simulink model "Boat_sim_HeadingHold"  (Simulink 7.5)
settings: Solver=FixedStepDiscrete  StartTime=0.0  StopTime=1000  FixedStep=.01  RelTol=1e-3
InitFcn:
  | boat_constants
values from neighbouring files (symbols this model uses):
  C_d_sea_surge = 340    [boat_constants.m]
  d_prop = .4572    (= 0.4572)    [boat_constants.m]
  figure8_waypoints = int32([ ... (first row only)    [boat_constants.m]
  K_t = 0.5    [boat_constants.m]
  mass = 550    [boat_constants.m]
  OC2max = 49999    [boat_constants.m]    (also in simulation_constants.m)
  phi_0 = 0    [boat_constants.m]    (also in simulation_constants.m)
  rho_w = 1.03e3    (= 1030)    [boat_constants.m]
  sampling_waypoints = int32([ ... (first row only)    [boat_constants.m]
  T_step = 0.01    [boat_constants.m]    (also in common.m)
  test_waypoints = int32([ ... (first row only)    [boat_constants.m]
  wheelbase = 3.27    [boat_constants.m]
undefined symbols (not defined in the file or in its folder): clock, DiscIntNeverNeededParam, Earth, WGS84
libraries: simulink x24, uSimLib x6, instrumentlib x2, aerolibconvert2 x2, aerolibtransform2 x1, aerolibanimutils x1, simulink_need_slupdate x1
(part 2 of 2)

== system Boat_sim_HeadingHold/Subsystem/Map from [347:655] to [0.7854:-0.7854] ==
  In1 : Inport
  Bias1 : Bias  Bias=-501
  Data Type Conversion : DataTypeConversion  OutDataTypeMode=single  OutDataType=fixdt(1, 16)  OutScaling=2^0  OutDataTypeStr=single
  Gain : Gain  Gain=-1/196  ParameterDataType=fixdt(1, 16)  ParameterScaling=2^0  OutDataType=fixdt(1, 16)  OutScaling=2^0
  Out1 : Outport
  wires:
  In1/1 -> Data Type Conversion/1
  Gain/1 -> Out1/1
  Bias1/1 -> Gain/1
  Data Type Conversion/1 -> Bias1/1

== system Boat_sim_HeadingHold/Plant/Actuator Dynamics/Enabled Subsystem ==
  note: Map from 0,1 to -.02,.02
  In1 : Inport  OutDataType=fixdt(1, 16)  OutScaling=2^0
  Enable : EnablePort
  Bias : Bias  Bias=-1
  Data Type Conversion3 : DataTypeConversion  OutDataTypeMode=single  OutDataType=sfix(16)  OutScaling=2^0  OutDataTypeStr=single
  Gain : Gain  Gain=2  ParameterDataType=fixdt(1, 16)  ParameterScaling=2^0  OutDataTypeMode=double  OutDataType=fixdt(1, 16)  OutScaling=2^0  OutDataTypeStr=double
  Gain1 : Gain  Gain=.05  ParameterDataType=fixdt(1, 16)  ParameterScaling=2^0  OutDataType=fixdt(1, 16)  OutScaling=2^0
  Out1 : Outport  OutDataType=fixdt(1, 16)  OutScaling=2^0
  wires:
  In1/1 -> Data Type Conversion3/1
  Gain/1 -> Bias/1
  Bias/1 -> Gain1/1
  Gain1/1 -> Out1/1
  Data Type Conversion3/1 -> Gain/1

== system Boat_sim_HeadingHold/Plant/Actuator Dynamics/Second Order Linear Actuator1 ==
  Ac_dem : Inport  OutDataType=sfix(16)  OutScaling=2^0
  2*zeta * wn : Gain  Gain=2.0 * z_fin* wn_fin  ParameterDataType=sfix(16)  ParameterScaling=2^0  OutDataType=sfix(16)  OutScaling=2^0  SaturateOnIntegerOverflow=on  OutDataTypeStr=Inherit: Same as input  ParamDataTypeStr=Inherit: Same as input
  Discrete-Time Integrator1 : DiscreteIntegrator  SampleTime=-1  OutDataType=fixdt(1, 16)  OutScaling=2^0  UpperSaturationLimit=1  LowerSaturationLimit=-1  ICPrevOutput=DiscIntNeverNeededParam  ICPrevScaledInput=DiscIntNeverNeededParam
  Discrete-Time Integrator2 : DiscreteIntegrator  SampleTime=-1  OutDataType=fixdt(1, 16)  OutScaling=2^0  UpperSaturationLimit=1  LowerSaturationLimit=-1  ICPrevOutput=DiscIntNeverNeededParam  ICPrevScaledInput=DiscIntNeverNeededParam
  Sum2 : Sum  Inputs=|+-  OutDataType=sfix(16)  OutScaling=2^0  SaturateOnIntegerOverflow=on  InputSameDT=on  OutDataTypeStr=Inherit: Same as first input
  Sum3 : Sum  Inputs=|+-  OutDataType=sfix(16)  OutScaling=2^0  SaturateOnIntegerOverflow=on  InputSameDT=on  OutDataTypeStr=Inherit: Same as first input
  wn^2 : Gain  Gain=wn_fin* wn_fin  ParameterDataType=sfix(16)  ParameterScaling=2^0  OutDataType=sfix(16)  OutScaling=2^0  SaturateOnIntegerOverflow=on  OutDataTypeStr=Inherit: Same as input  ParamDataTypeStr=Inherit: Same as input
  Ac_ac : Outport  OutDataType=sfix(16)  OutScaling=2^0  InitialOutput=0
  wires:
  Discrete-Time Integrator1/1 -> Ac_ac/1, Sum3/2
  wn^2/1 -> Sum2/1
  Sum2/1 -> Discrete-Time Integrator2/1
  Discrete-Time Integrator2/1 -> 2*zeta * wn/1, Discrete-Time Integrator1/1
  2*zeta * wn/1 -> Sum2/2
  Ac_dem/1 -> Sum3/1
  Sum3/1 -> wn^2/1

== system Boat_sim_HeadingHold/Plant/Actuator Dynamics/Second Order Linear Actuator2 ==
  Ac_dem : Inport  OutDataType=sfix(16)  OutScaling=2^0
  2*zeta * wn : Gain  Gain=2.0 * z_fin* wn_fin  ParameterDataType=sfix(16)  ParameterScaling=2^0  OutDataType=sfix(16)  OutScaling=2^0  SaturateOnIntegerOverflow=on  OutDataTypeStr=Inherit: Same as input  ParamDataTypeStr=Inherit: Same as input
  Discrete-Time Integrator1 : DiscreteIntegrator  SampleTime=-1  OutDataType=fixdt(1, 16)  OutScaling=2^0  UpperSaturationLimit=1  LowerSaturationLimit=-1  ICPrevOutput=DiscIntNeverNeededParam  ICPrevScaledInput=DiscIntNeverNeededParam
  Discrete-Time Integrator2 : DiscreteIntegrator  SampleTime=-1  OutDataType=fixdt(1, 16)  OutScaling=2^0  UpperSaturationLimit=1  LowerSaturationLimit=-1  ICPrevOutput=DiscIntNeverNeededParam  ICPrevScaledInput=DiscIntNeverNeededParam
  Sum2 : Sum  Inputs=|+-  OutDataType=sfix(16)  OutScaling=2^0  SaturateOnIntegerOverflow=on  InputSameDT=on  OutDataTypeStr=Inherit: Same as first input
  Sum3 : Sum  Inputs=|+-  OutDataType=sfix(16)  OutScaling=2^0  SaturateOnIntegerOverflow=on  InputSameDT=on  OutDataTypeStr=Inherit: Same as first input
  wn^2 : Gain  Gain=wn_fin* wn_fin  ParameterDataType=sfix(16)  ParameterScaling=2^0  OutDataType=sfix(16)  OutScaling=2^0  SaturateOnIntegerOverflow=on  OutDataTypeStr=Inherit: Same as input  ParamDataTypeStr=Inherit: Same as input
  Ac_ac : Outport  OutDataType=sfix(16)  OutScaling=2^0  InitialOutput=0
  wires:
  Discrete-Time Integrator1/1 -> Ac_ac/1, Sum3/2
  wn^2/1 -> Sum2/1
  Sum2/1 -> Discrete-Time Integrator2/1
  Discrete-Time Integrator2/1 -> 2*zeta * wn/1, Discrete-Time Integrator1/1
  2*zeta * wn/1 -> Sum2/2
  Ac_dem/1 -> Sum3/1
  Sum3/1 -> wn^2/1

== system Boat_sim_HeadingHold/Plant/Actuator Dynamics/Second Order Linear Actuator3 ==
  Ac_dem : Inport  OutDataType=sfix(16)  OutScaling=2^0
  2*zeta * wn : Gain  Gain=2.0 * z_fin* wn_fin  ParameterDataType=sfix(16)  ParameterScaling=2^0  OutDataType=sfix(16)  OutScaling=2^0  SaturateOnIntegerOverflow=on  OutDataTypeStr=Inherit: Same as input  ParamDataTypeStr=Inherit: Same as input
  Discrete-Time Integrator1 : DiscreteIntegrator  SampleTime=-1  OutDataType=fixdt(1, 16)  OutScaling=2^0  UpperSaturationLimit=1  LowerSaturationLimit=-1  ICPrevOutput=DiscIntNeverNeededParam  ICPrevScaledInput=DiscIntNeverNeededParam
  Discrete-Time Integrator2 : DiscreteIntegrator  SampleTime=-1  OutDataType=fixdt(1, 16)  OutScaling=2^0  UpperSaturationLimit=1  LowerSaturationLimit=-1  ICPrevOutput=DiscIntNeverNeededParam  ICPrevScaledInput=DiscIntNeverNeededParam
  Sum2 : Sum  Inputs=|+-  OutDataType=sfix(16)  OutScaling=2^0  SaturateOnIntegerOverflow=on  InputSameDT=on  OutDataTypeStr=Inherit: Same as first input
  Sum3 : Sum  Inputs=|+-  OutDataType=sfix(16)  OutScaling=2^0  SaturateOnIntegerOverflow=on  InputSameDT=on  OutDataTypeStr=Inherit: Same as first input
  wn^2 : Gain  Gain=wn_fin* wn_fin  ParameterDataType=sfix(16)  ParameterScaling=2^0  OutDataType=sfix(16)  OutScaling=2^0  SaturateOnIntegerOverflow=on  OutDataTypeStr=Inherit: Same as input  ParamDataTypeStr=Inherit: Same as input
  Ac_ac : Outport  OutDataType=sfix(16)  OutScaling=2^0  InitialOutput=0
  wires:
  Discrete-Time Integrator1/1 -> Ac_ac/1, Sum3/2
  wn^2/1 -> Sum2/1
  Sum2/1 -> Discrete-Time Integrator2/1
  Discrete-Time Integrator2/1 -> 2*zeta * wn/1, Discrete-Time Integrator1/1
  2*zeta * wn/1 -> Sum2/2
  Ac_dem/1 -> Sum3/1
  Sum3/1 -> wn^2/1

== system Boat_sim_HeadingHold/Plant/Actuator Dynamics/Subsystem ==
  note: This block stores the throttle speed. As the speed is only set intermittently,
      | the speed is saved to memory and constrantly output. It is only updated when
      | a properly packaged CAN message is delivered based on its ID and the trigger
      | bit.
  In1 : Inport
  Bus Selector2 : BusSelector  OutputSignals=identifier,trigger,data
  Data Store Memory : DataStoreMemory  DataStoreName=throttle_speed  WriteAfterWriteMsg=warning  WriteAfterReadMsg=warning  DataType=double  OutDataType=fixdt(1, 16)  OutScaling=2^0  OutDataTypeStr=double
  Data Store Read : DataStoreRead  Priority=2  DataStoreName=throttle_speed  SampleTime=T_step
  Data Type Conversion : DataTypeConversion  OutDataTypeMode=uint32  OutDataType=fixdt(1, 16)  OutScaling=2^0  OutDataTypeStr=uint32  RndMeth=Simplest
  If : If  NumInputs=2  IfExpression=u1 == hex2dec('301')  ShowElse=off
  If Action Subsystem : Subsystem  Priority=1  TreatAsAtomicUnit=on
  Scope1 : Scope
      settings: YMin=971.85  YMax=1074.15  SaveName=ScopeData2
  To Workspace : ToWorkspace  VariableName=t_data  SampleTime=-1  SaveFormat=Structure
  Out1 : Outport
  wires:
  In1/1 -> Bus Selector2/1
  Data Store Read/1 -> Out1/1, Scope1/1
  Bus Selector2/1 -> If/1  "<identifier>"
  Bus Selector2/2 -> Data Type Conversion/1  "<trigger>"
  If/1 -> If Action Subsystem/Action
  Bus Selector2/3 -> If Action Subsystem/1(In1), To Workspace/1  "<data>"
  Data Type Conversion/1 -> If/2

== system Boat_sim_HeadingHold/Plant/Actuator Dynamics/Subsystem1 ==
  note: This block simulates the stepper motor driver board logic for stepping the motor.
      | The enable line must be low, it's active low, and a pulse train must be received. As
      | the enable line is always low to provide holding torque, the lines specifying a pulse
      | train must are therefore checked to confirm that the rudder should be moving. The
      | exact values of both the up and period signals are unimportant, so they're just
      | compared to zero.
  e : Inport
  u : Inport  Port=2
  p : Inport  Port=3
  Compare To Zero : simulink/Logic and Bit Operations/Compare To Zero  SystemSampleTime=-1  relop=~=  LogicOutDataTypeMode=boolean
  Compare To Zero1 : simulink/Logic and Bit Operations/Compare To Zero  SystemSampleTime=-1  relop=~=  LogicOutDataTypeMode=boolean
  Logical Operator : Logic  Operator=NOT  AllPortsSameDT=off  OutDataTypeMode=boolean  LogicDataType=fixdt(0, 8)  OutDataTypeStr=boolean
  Logical Operator1 : Logic  Inputs=3  AllPortsSameDT=off  OutDataTypeMode=boolean  LogicDataType=fixdt(0, 8)  OutDataTypeStr=boolean
  Out1 : Outport
  wires:
  e/1 -> Logical Operator/1
  Logical Operator1/1 -> Out1/1
  p/1 -> Compare To Zero/1
  Compare To Zero/1 -> Logical Operator1/3
  Compare To Zero1/1 -> Logical Operator1/2
  u/1 -> Compare To Zero1/1
  Logical Operator/1 -> Logical Operator1/1

== system Boat_sim_HeadingHold/Plant/Generate sensor data from actuator position/Map from +-.7854 to [347:655] ==
  In1 : Inport
  Bias1 : Bias  Bias=501
  Data Type Conversion : DataTypeConversion  OutDataTypeMode=uint16  OutDataType=fixdt(1, 16)  OutScaling=2^0  OutDataTypeStr=uint16
  Gain1 : Gain  Gain=-196  ParameterDataType=fixdt(1, 16)  ParameterScaling=2^0  OutDataType=fixdt(1, 16)  OutScaling=2^0
  Out1 : Outport
  wires:
  Bias1/1 -> Data Type Conversion/1
  In1/1 -> Gain1/1
  Data Type Conversion/1 -> Out1/1
  Gain1/1 -> Bias1/1

== system Boat_sim_HeadingHold/Plant/Generate sensor data from actuator position/Map from -1..1 to -1023..1023 ==
  In1 : Inport
  Data Type Conversion : DataTypeConversion  OutDataTypeMode=int16  OutDataType=fixdt(1, 16)  OutScaling=2^0  OutDataTypeStr=int16  RndMeth=Simplest
  Gain : Gain  Gain=1023  ParameterDataType=fixdt(1, 16)  ParameterScaling=2^0  OutDataType=fixdt(1, 16)  OutScaling=2^0
  Out1 : Outport
  wires:
  Gain/1 -> Data Type Conversion/1
  In1/1 -> Gain/1
  Data Type Conversion/1 -> Out1/1

== system Boat_sim_HeadingHold/Plant/Generate sensor data from actuator position/Map from -1..1 to 620..313 ==
  In1 : Inport
  Bias : Bias  Bias=466.5
  Data Type Conversion : DataTypeConversion  OutDataTypeMode=uint16  OutDataType=fixdt(1, 16)  OutScaling=2^0  OutDataTypeStr=uint16
  Gain : Gain  Gain=-153.5  ParameterDataType=fixdt(1, 16)  ParameterScaling=2^0  OutDataType=fixdt(1, 16)  OutScaling=2^0
  Out1 : Outport
  wires:
  Data Type Conversion/1 -> Out1/1
  In1/1 -> Gain/1
  Bias/1 -> Data Type Conversion/1
  Gain/1 -> Bias/1

== system Boat_sim_HeadingHold/Subsystem/Autonomous Controller/Ballast Command ==
  Bus Creator : BusCreator  Inputs=2
  Constant : Constant  Value=0  OutDataTypeMode=boolean  OutDataType=fixdt(1, 16)  OutScaling=2^0  OutDataTypeStr=boolean
  Constant1 : Constant  Value=0  OutDataTypeMode=boolean  OutDataType=fixdt(1, 16)  OutScaling=2^0  OutDataTypeStr=boolean
  c_ballast : Outport
  wires:
  Constant1/1 -> Bus Creator/2  "direction"
  Constant/1 -> Bus Creator/1  "enable"
  Bus Creator/1 -> c_ballast/1

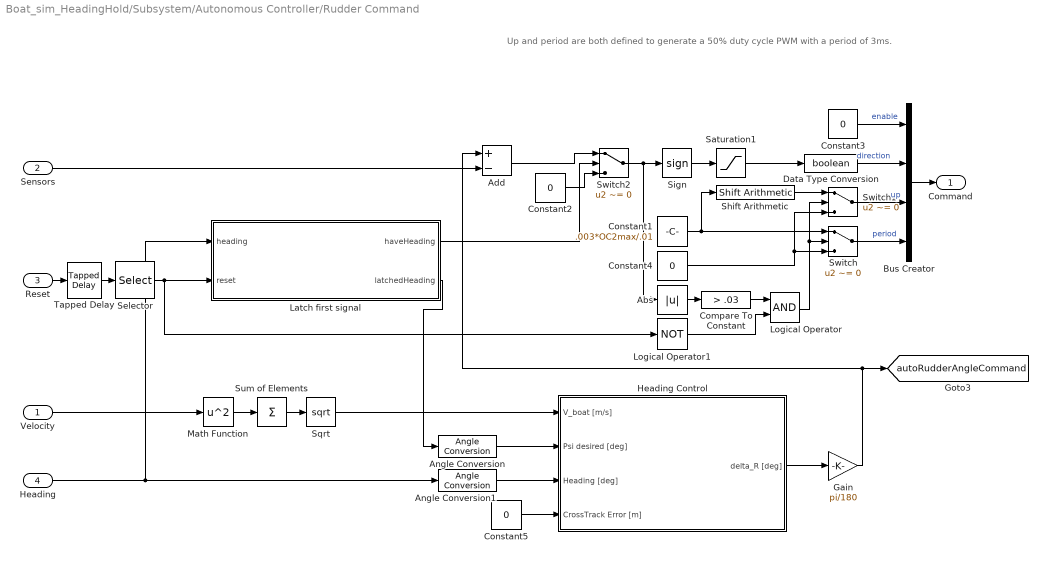
== system Boat_sim_HeadingHold/Subsystem/Autonomous Controller/Rudder Command ==
  note: Up and period are both defined to generate a 50% duty cycle PWM with
      | a period of 3ms.
  Velocity : Inport
  Sensors : Inport  Port=2
  Reset : Inport  Port=3
  Heading : Inport  Port=4
  Abs : Abs  OutDataType=fixdt(1, 16)  OutScaling=2^0
  Add : Sum  Inputs=+-  OutDataType=fixdt(1, 16)  OutScaling=2^-10
  Angle Conversion : uSimLib/Conversions/Angle Conversion  SystemSampleTime=-1  iu=rad  ou=deg
  Angle Conversion1 : uSimLib/Conversions/Angle Conversion  SystemSampleTime=-1  iu=rad  ou=deg
  Bus Creator : BusCreator
  Compare To Constant : simulink/Logic and Bit Operations/Compare To Constant  SystemSampleTime=-1  relop=>  const=.03  LogicOutDataTypeMode=boolean
  Constant1 : Constant  Value=.003*OC2max/.01  OutDataTypeMode=uint16  OutDataType=sfix(16)  OutScaling=2^0  OutDataTypeStr=uint16
  Constant2 : Constant  Value=0  OutDataTypeMode=single  OutDataType=sfix(16)  OutScaling=2^0  OutDataTypeStr=single
  Constant3 : Constant  Value=0  OutDataTypeMode=boolean  OutDataType=sfix(16)  OutScaling=2^0  OutDataTypeStr=boolean
  Constant4 : Constant  Value=0  OutDataTypeMode=uint16  OutDataType=sfix(16)  OutScaling=2^0  OutDataTypeStr=uint16
  Constant5 : Constant  Value=0  OutDataTypeMode=uint8  OutDataType=sfix(16)  OutScaling=2^0  OutDataTypeStr=uint8
  Data Type Conversion : DataTypeConversion  OutDataTypeMode=boolean  OutDataType=fixdt(1, 16)  OutScaling=2^0  OutDataTypeStr=boolean  RndMeth=Simplest
  Gain : Gain  Gain=pi/180  ParameterDataType=fixdt(1, 16)  ParameterScaling=2^0  OutDataTypeMode=single  OutDataType=fixdt(1, 16)  OutScaling=2^0  OutDataTypeStr=single
  Heading Control : Subsystem
  Latch first signal : Stateflow chart  TreatAsAtomicUnit=on
  Logical Operator : Logic  AllPortsSameDT=off  OutDataTypeMode=boolean  LogicDataType=fixdt(0, 8)  OutDataTypeStr=boolean
  Logical Operator1 : Logic  Operator=NOT  Inputs=1  AllPortsSameDT=off  OutDataTypeMode=boolean  LogicDataType=fixdt(0, 8)  OutDataTypeStr=boolean
  Math Function : Math  Operator=square  OutDataType=fixdt(1, 16)  OutScaling=2^0  SaturateOnIntegerOverflow=on
  Saturation1 : Saturate  UpperLimit=1  LowerLimit=0  OutDataTypeStr=Inherit: Inherit via back propagation
  Selector : Selector  InputPortWidth=100  IndexOptions=Index vector (dialog)  Indices=1  OutputSizes=1
  Shift Arithmetic : simulink/Logic and Bit Operations/Shift Arithmetic  SystemSampleTime=-1  nBitShiftRight=1  nBinPtShiftRight=0
  Sign : Signum
  Sqrt : Sqrt  OutDataTypeMode=single  OutDataTypeStr=single  SaturateOnIntegerOverflow=on
  Sum of Elements : Sum  Inputs=+  OutDataTypeMode=single  OutDataType=fixdt(1, 16)  OutScaling=2^-10  OutDataTypeStr=single
  Switch : Switch  Criteria=u2 ~= 0  OutDataType=fixdt(1, 16)  OutScaling=2^0
  Switch1 : Switch  Criteria=u2 ~= 0  OutDataType=fixdt(1, 16)  OutScaling=2^0
  Switch2 : Switch  Criteria=u2 ~= 0  OutDataType=fixdt(1, 16)  OutScaling=2^0
  Tapped Delay : simulink/Discrete/Tapped Delay  vinit=0  samptime=-1  NumDelays=100  DelayOrder=Oldest  includeCurrent=off
  Command : Outport
  tag scope: autoRudderAngleCommand=global
  wires:
  Angle Conversion1/1 -> Heading Control/3(Heading [deg])
  Gain/1 -> Add/1, [autoRudderAngleCommand]
  Heading Control/1(delta_R [deg]) -> Gain/1
  Sum of Elements/1 -> Sqrt/1
  Math Function/1 -> Sum of Elements/1
  Sqrt/1 -> Heading Control/1(V_boat [m/s])
  Constant5/1 -> Heading Control/4(CrossTrack Error [m])
  Heading/1 -> Angle Conversion1/1, Latch first signal/1(heading)
  Logical Operator1/1 -> Logical Operator/2
  Logical Operator/1 -> Switch1/2, Switch/2
  Compare To Constant/1 -> Logical Operator/1
  Reset/1 -> Tapped Delay/1
  Constant4/1 -> Switch1/3, Switch/3
  Switch1/1 -> Bus Creator/3  "up"
  Switch/1 -> Bus Creator/4  "period"
  Shift Arithmetic/1 -> Switch1/1
  Abs/1 -> Compare To Constant/1
  Constant1/1 -> Switch/1, Shift Arithmetic/1
  Constant3/1 -> Bus Creator/1  "enable"
  Velocity/1 -> Math Function/1
  Sign/1 -> Saturation1/1
  Saturation1/1 -> Data Type Conversion/1
  Bus Creator/1 -> Command/1
  Sensors/1 -> Add/2
  Data Type Conversion/1 -> Bus Creator/2  "direction"
  Latch first signal/2(latchedHeading) -> Angle Conversion/1
  Latch first signal/1(haveHeading) -> Switch2/2
  Add/1 -> Switch2/1
  Constant2/1 -> Switch2/3
  Switch2/1 -> Sign/1, Abs/1
  Angle Conversion/1 -> Heading Control/2(Psi desired [deg])
  Tapped Delay/1 -> Selector/1
  Selector/1 -> Logical Operator1/1, Latch first signal/2(reset)

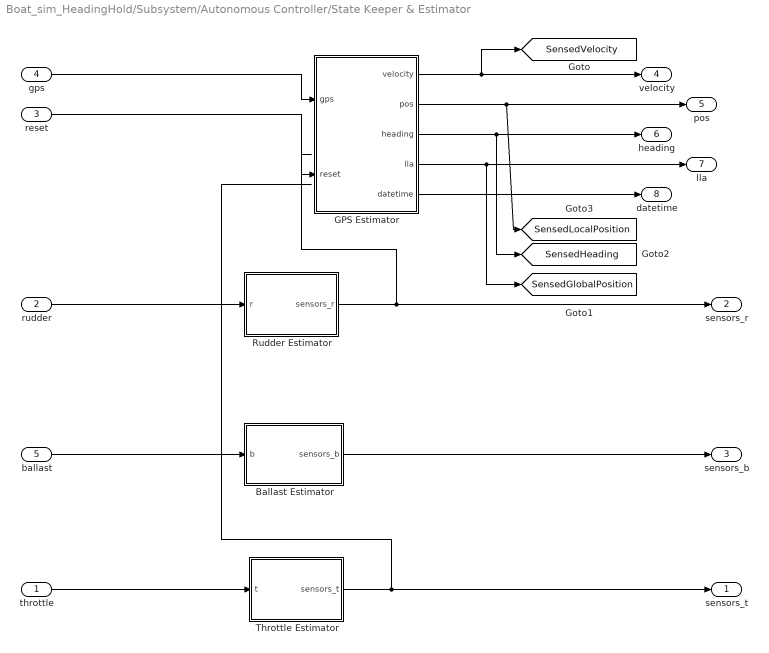
== system Boat_sim_HeadingHold/Subsystem/Autonomous Controller/State Keeper & Estimator ==
  throttle : Inport
  rudder : Inport  Port=2
  reset : Inport  Port=3
  gps : Inport  Port=4
  ballast : Inport  Port=5
  Ballast Estimator : Subsystem
  GPS Estimator : Subsystem
  Rudder Estimator : Subsystem
  Throttle Estimator : Subsystem
  sensors_t : Outport
  sensors_r : Outport  Port=2
  sensors_b : Outport  Port=3
  velocity : Outport  Port=4
  pos : Outport  Port=5
  heading : Outport  Port=6
  lla : Outport  Port=7
  datetime : Outport  Port=8
  tag scope: SensedGlobalPosition=global, SensedHeading=global, SensedLocalPosition=global, SensedVelocity=global
  wires:
  Throttle Estimator/1(sensors_t) -> sensors_t/1
  Ballast Estimator/1(sensors_b) -> sensors_b/1
  Rudder Estimator/1(sensors_r) -> sensors_r/1
  GPS Estimator/5(datetime) -> datetime/1
  GPS Estimator/4(lla) -> lla/1, [SensedGlobalPosition]
  GPS Estimator/3(heading) -> [SensedHeading], heading/1
  GPS Estimator/2(pos) -> [SensedLocalPosition], pos/1
  gps/1 -> GPS Estimator/1(gps)
  GPS Estimator/1(velocity) -> [SensedVelocity], velocity/1
  reset/1 -> GPS Estimator/2(reset)
  throttle/1 -> Throttle Estimator/1(t)
  ballast/1 -> Ballast Estimator/1(b)
  rudder/1 -> Rudder Estimator/1(r)

== system Boat_sim_HeadingHold/Subsystem/Autonomous Controller/Throttle Command ==
  sensors : Inport
  reset : Inport  Port=2
  Bus Creator : BusCreator
  Constant1 : Constant  Value=0  OutDataTypeMode=int16  OutDataType=sfix(16)  OutScaling=2^0  OutDataTypeStr=int16
  Constant5 : Constant  Value=1000  OutDataTypeMode=int16  OutDataType=sfix(16)  OutScaling=2^0  OutDataTypeStr=int16
  Mux Everything : Subsystem
  Switch : Switch  Criteria=u2 > Threshold  OutDataType=fixdt(1, 16)  OutScaling=2^0
  Terminator : Terminator
  Trigger Events : Subsystem
  command : Outport  OutDataType=sfix(16)  OutScaling=2^0
  tag scope: autoThrottleCommand=global
  wires:
  Constant5/1 -> Switch/3
  Constant1/1 -> Switch/1
  Switch/1 -> Trigger Events/1(RC Throttle), Mux Everything/4(Throttle), [autoThrottleCommand]
  Mux Everything/4(trig) -> Bus Creator/4  "trigger"
  Mux Everything/3(size) -> Bus Creator/3  "size"
  Mux Everything/2(data) -> Bus Creator/2  "data"
  Mux Everything/1(iden) -> Bus Creator/1  "identifier"
  reset/1 -> Switch/2, Trigger Events/2(Reset)
  Trigger Events/2(Disable) -> Mux Everything/2(disable)
  Trigger Events/3(Enable) -> Mux Everything/3(enable)
  Trigger Events/1(Change Speed) -> Mux Everything/1(speed)
  Bus Creator/1 -> command/1
  sensors/1 -> Terminator/1

== system Boat_sim_HeadingHold/Plant/Actuator Dynamics/Subsystem/If Action Subsystem ==
  In1 : Inport  OutDataType=fixdt(1, 16)  OutScaling=2^0
  Action Port : ActionPort  ActionType=then
  Bitwise Operator : simulink/Logic and Bit Operations/Bitwise Operator  logicop=OR  UseBitMask=off  NumInputPorts=2  BitMask=bin2dec('11011001')  BitMaskRealWorld=Stored Integer
  Data Store Write : DataStoreWrite  DataStoreName=throttle_speed  SampleTime=-1
  Data Type Conversion : DataTypeConversion  OutDataTypeMode=uint16  OutDataType=fixdt(1, 16)  OutScaling=2^0  OutDataTypeStr=uint16  ConvertRealWorld=Stored Integer (SI)
  Data Type Conversion2 : DataTypeConversion  OutDataTypeMode=double  OutDataType=sfix(16)  OutScaling=2^0  OutDataTypeStr=double  LockScale=on
  Demux : Demux  Outputs=2
  Gain : Gain  Gain=1/1023  ParameterDataType=fixdt(1, 16)  ParameterScaling=2^0  OutDataType=fixdt(1, 16)  OutScaling=2^0
  Selector2 : Selector  InputPortWidth=6  IndexOptions=Index vector (dialog)  Indices=[4 3]  OutputSizes=1
  Shift Arithmetic : simulink/Logic and Bit Operations/Shift Arithmetic  SystemSampleTime=-1  nBitShiftRight=-8  nBinPtShiftRight=0
  wires:
  In1/1 -> Selector2/1
  Data Type Conversion2/1 -> Gain/1
  Gain/1 -> Data Store Write/1
  Selector2/1 -> Data Type Conversion/1
  Bitwise Operator/1 -> Data Type Conversion2/1
  Data Type Conversion/1 -> Demux/1
  Demux/1 -> Bitwise Operator/1
  Demux/2 -> Shift Arithmetic/1
  Shift Arithmetic/1 -> Bitwise Operator/2

== system Boat_sim_HeadingHold/Subsystem/Autonomous Controller/Rudder Command/Heading Control ==
  note: Heading Error
  V_boat [m/s] : Inport  OutDataType=sfix(16)  OutScaling=2^0
  Psi desired [deg] : Inport  Port=2  OutDataType=sfix(16)  OutScaling=2^0
  Heading [deg] : Inport  Port=3  OutDataType=sfix(16)  OutScaling=2^0
  CrossTrack Error [m] : Inport  Port=4  OutDataType=sfix(16)  OutScaling=2^0
  Abs : Abs
  Angle Conversion : aerolibconvert2/Angle Conversion  SystemSampleTime=-1  IU=deg  OU=rad
  Angle Conversion1 : aerolibconvert2/Angle Conversion  SystemSampleTime=-1  IU=rad  OU=deg
  Constant : Constant  OutDataType=sfix(16)  OutScaling=2^0
  Divide : Product  Inputs=*/  OutDataType=sfix(16)  OutScaling=2^-10
  Fcn2 : Fcn  Expr=(u<-180)*360 + u + (u>180)*(-360)
  Kpsi : Gain  ParameterDataType=sfix(16)  ParameterScaling=2^0  OutDataType=sfix(16)  OutScaling=2^0
  MinMax : MinMax  Function=max  Inputs=2  OutDataType=sfix(16)  OutScaling=2^0
  Product : Product  OutDataType=sfix(16)  OutScaling=2^0  RndMeth=Zero
  Saturation : Saturate  UpperLimit=45  LowerLimit=-45
  Scope : Scope
      settings: SaveName=ScopeData4
  Sign : Signum
  Sum : Sum  Inputs=-+|  OutDataType=sfix(16)  OutScaling=2^0
  Terminator : Terminator
  delta_R [deg] : Outport  OutDataType=sfix(16)  OutScaling=2^0
  wires:
  Fcn2/1 -> Angle Conversion/1, Scope/1
  Angle Conversion/1 -> Kpsi/1
  V_boat [m/s]/1 -> Abs/1, Sign/1
  Product/1 -> Angle Conversion1/1
  Kpsi/1 -> Product/2
  Sign/1 -> Product/1
  Angle Conversion1/1 -> Divide/1
  Divide/1 -> Saturation/1
  Abs/1 -> MinMax/1
  Constant/1 -> MinMax/2
  Saturation/1 -> delta_R [deg]/1
  MinMax/1 -> Divide/2
  CrossTrack Error [m]/1 -> Terminator/1
  Psi desired [deg]/1 -> Sum/1
  Heading [deg]/1 -> Sum/2
  Sum/1 -> Fcn2/1

== system Boat_sim_HeadingHold/Subsystem/Autonomous Controller/State Keeper & Estimator/Ballast Estimator ==
  b : Inport
  Bus Selector1 : BusSelector  OutputSignals=position
  sensors_b : Outport
  wires:
  Bus Selector1/1 -> sensors_b/1  "<position>"
  b/1 -> Bus Selector1/1

== system Boat_sim_HeadingHold/Subsystem/Autonomous Controller/State Keeper & Estimator/GPS Estimator ==
  gps : Inport
  reset : Inport  Port=2  OutDataType=fixdt(1, 16)  OutScaling=2^0
  Add : Sum  OutDataType=fixdt(1, 16)  OutScaling=2^-10
  Bus Selector1 : BusSelector  OutputSignals=latitude,longitude,altitude,newData
  Calculate local position via velocity integral between true GPS updates : Stateflow chart  TreatAsAtomicUnit=on
  Discrete-Time Integrator4 : DiscreteIntegrator  ExternalReset=level  SampleTime=-1  OutDataType=fixdt(1, 16)  OutScaling=2^0  ICPrevOutput=DiscIntNeverNeededParam  ICPrevScaledInput=DiscIntNeverNeededParam
  Mux1 : Mux  Inputs=3
  Subsystem : Subsystem
  velocity : Outport
  pos : Outport  Port=2
  heading : Outport  Port=3
  lla : Outport  Port=4
  datetime : Outport  Port=5
  wires:
  Subsystem/1(velocity) -> velocity/1, Discrete-Time Integrator4/1
  Calculate local position via velocity integral between true GPS updates/1(localPosition) -> Add/1
  Calculate local position via velocity integral between true GPS updates/2(resetIntegrator) -> Discrete-Time Integrator4/2
  Mux1/1 -> Calculate local position via velocity integral between true GPS updates/1(latLonAlt)
  Bus Selector1/4 -> Calculate local position via velocity integral between true GPS updates/2(newData)  "<newData>"
  Bus Selector1/3 -> Mux1/3  "<altitude>"
  Bus Selector1/2 -> Mux1/2  "<longitude>"
  Bus Selector1/1 -> Mux1/1  "<latitude>"
  Add/1 -> pos/1
  Discrete-Time Integrator4/1 -> Add/2
  reset/1 -> Calculate local position via velocity integral between true GPS updates/3(reset)
  Subsystem/4(time) -> datetime/1
  Subsystem/3(pos) -> lla/1
  gps/1 -> Bus Selector1/1, Subsystem/1(gps)
  Subsystem/2(heading) -> heading/1

== system Boat_sim_HeadingHold/Subsystem/Autonomous Controller/State Keeper & Estimator/Rudder Estimator ==
  r : Inport
  sensors_r : Outport
  wires:
  r/1 -> sensors_r/1

== system Boat_sim_HeadingHold/Subsystem/Autonomous Controller/State Keeper & Estimator/Throttle Estimator ==
  t : Inport
  sensors_t : Outport
  wires:
  t/1 -> sensors_t/1

== system Boat_sim_HeadingHold/Subsystem/Autonomous Controller/Throttle Command/Mux Everything ==
  speed : Inport  OutDataType=sfix(16)  OutScaling=2^0
  disable : Inport  Port=2  OutDataType=sfix(16)  OutScaling=2^0
  enable : Inport  Port=3  OutDataType=sfix(16)  OutScaling=2^0
  Throttle : Inport  Port=4  OutDataType=sfix(16)  OutScaling=2^0
  0x300 : Constant  Value=768  OutDataTypeMode=uint32  OutDataType=sfix(16)  OutScaling=2^0  OutDataTypeStr=uint32
  0x301 : Constant  Value=769  OutDataTypeMode=uint32  OutDataType=sfix(16)  OutScaling=2^0  OutDataTypeStr=uint32
  Build speed command : Subsystem
  Disable motor : Constant  Value=[0 0 0 0 64 0]  OutDataTypeMode=uint8  OutDataType=sfix(16)  OutScaling=2^0  OutDataTypeStr=uint8
  Enable motor : Constant  Value=[0 0 0 0 32 0]  OutDataTypeMode=uint8  OutDataType=sfix(16)  OutScaling=2^0  OutDataTypeStr=uint8
  Logical Operator1 : Logic  Operator=OR  AllPortsSameDT=off  OutDataTypeMode=boolean  OutDataTypeStr=boolean
  Message Length1 : Probe  ProbeSampleTime=off  ProbeComplexSignal=off  ProbeWidthDataType=uint8
  Multiport Switch : MultiPortSwitch  zeroidx=off
  Multiport Switch1 : MultiPortSwitch  zeroidx=off
  Select data packet : Stateflow chart  TreatAsAtomicUnit=on
  Switch : Switch  Criteria=u2 ~= 0
  iden : Outport  OutDataType=sfix(16)  OutScaling=2^0
  data : Outport  Port=2  OutDataType=sfix(16)  OutScaling=2^0
  size : Outport  Port=3  OutDataType=sfix(16)  OutScaling=2^0
  trig : Outport  Port=4  OutDataType=sfix(16)  OutScaling=2^0
  wires:
  Build speed command/1(msg) -> Multiport Switch/4
  speed/1 -> Multiport Switch1/4
  Multiport Switch1/1 -> trig/1
  Select data packet/1(y) -> Multiport Switch1/1, Multiport Switch/1
  Logical Operator1/1 -> Switch/2
  enable/1 -> Multiport Switch1/3, Select data packet/2(en), Logical Operator1/2
  disable/1 -> Multiport Switch1/2, Select data packet/1(dis), Logical Operator1/1
  Switch/1 -> iden/1
  0x301/1 -> Switch/3
  0x300/1 -> Switch/1
  Message Length1/1 -> size/1
  Multiport Switch/1 -> data/1, Message Length1/1
  Throttle/1 -> Build speed command/1(CC)
  Disable motor/1 -> Multiport Switch/2
  Enable motor/1 -> Multiport Switch/3

== system Boat_sim_HeadingHold/Subsystem/Autonomous Controller/Throttle Command/Trigger Events ==
  RC Throttle : Inport  OutDataType=sfix(16)  OutScaling=2^0
  Reset : Inport  Port=2  OutDataType=sfix(16)  OutScaling=2^0
  Data Type Conversion1 : DataTypeConversion  OutDataTypeMode=boolean  OutDataType=sfix(16)  OutScaling=2^0  OutDataTypeStr=boolean
  Data Type Conversion2 : DataTypeConversion  OutDataTypeMode=boolean  OutDataType=sfix(16)  OutScaling=2^0  OutDataTypeStr=boolean
  Data Type Conversion3 : DataTypeConversion  OutDataTypeMode=boolean  OutDataType=sfix(16)  OutScaling=2^0  OutDataTypeStr=boolean
  Detect Change : simulink/Logic and Bit Operations/Detect Change  SystemSampleTime=-1  vinit=0
  Detect Fall Nonpositive : simulink/Logic and Bit Operations/Detect Fall Nonpositive  SystemSampleTime=-1  vinit=0
  Detect Rise Positive : simulink/Logic and Bit Operations/Detect Rise Positive  SystemSampleTime=-1  vinit=0
  Shift Arithmetic : simulink/Logic and Bit Operations/Shift Arithmetic  SystemSampleTime=-1  nBitShiftRight=2  nBinPtShiftRight=0
  Weighted Moving Average : simulink_need_slupdate/Weighted Moving Average  mgainval=[.5 .5]  vinit=0.0  samptime=-1  OutDataTypeStr=Inherit: Inherit via back propagation  OutDataType=sfix(16)  OutScaling=2^-10  DoSatur=off  GainDataType=uint(16)  MatRadixGroup=Best Precision: Matrix-wise  GainScaling=2^-10
  Change Speed : Outport  OutDataType=sfix(16)  OutScaling=2^0
  Disable : Outport  Port=2  OutDataType=sfix(16)  OutScaling=2^0
  Enable : Outport  Port=3  OutDataType=sfix(16)  OutScaling=2^0
  wires:
  Data Type Conversion1/1 -> Disable/1
  Data Type Conversion2/1 -> Enable/1
  Data Type Conversion3/1 -> Change Speed/1
  Detect Rise Positive/1 -> Data Type Conversion1/1
  Detect Fall Nonpositive/1 -> Data Type Conversion2/1
  Reset/1 -> Detect Rise Positive/1, Detect Fall Nonpositive/1
  Shift Arithmetic/1 -> Weighted Moving Average/1
  Weighted Moving Average/1 -> Detect Change/1
  Detect Change/1 -> Data Type Conversion3/1
  RC Throttle/1 -> Shift Arithmetic/1

== system Boat_sim_HeadingHold/Subsystem/Autonomous Controller/State Keeper & Estimator/GPS Estimator/Subsystem ==
  note: Multiply by .51444 to
      | convert knots to m/s
  gps : Inport
  Angle Conversion : uSimLib/Conversions/Angle Conversion  SystemSampleTime=-1  iu=deg  ou=rad
  Bus Selector : BusSelector  OutputSignals=sog
  Bus Selector1 : BusSelector  OutputSignals=cog
  Constant : Constant  Value=0  OutDataTypeMode=single  OutDataType=fixdt(1, 16)  OutScaling=2^0  OutDataTypeStr=single
  Gain : Gain  Gain=.5144444  ParameterDataType=fixdt(1, 16)  ParameterScaling=2^0  OutDataType=fixdt(1, 16)  OutScaling=2^0
  Mux : Mux  Inputs=3
  Product : Product  OutDataTypeMode=single  OutDataType=fixdt(1, 16)  OutScaling=2^0  OutDataTypeStr=single  RndMeth=Zero
  Product1 : Product  OutDataTypeMode=single  OutDataType=fixdt(1, 16)  OutScaling=2^0  OutDataTypeStr=single  RndMeth=Zero
  Reorder : Subsystem
  Trigonometric Function : Trigonometry
  Trigonometric Function1 : Trigonometry  Operator=cos
  velocity : Outport
  heading : Outport  Port=2
  pos : Outport  Port=3
  time : Outport  Port=4
  wires:
  Gain/1 -> Product1/1, Product/1
  gps/1 -> Reorder/1(In1), Bus Selector/1, Bus Selector1/1
  Bus Selector1/1 -> Angle Conversion/1  "<cog>"
  Trigonometric Function/1 -> Product/2
  Trigonometric Function1/1 -> Product1/2
  Product1/1 -> Mux/1
  Product/1 -> Mux/2
  Constant/1 -> Mux/3
  Mux/1 -> velocity/1
  Angle Conversion/1 -> heading/1, Trigonometric Function/1, Trigonometric Function1/1
  Bus Selector/1 -> Gain/1  "<sog>"
  Reorder/1(pos) -> pos/1
  Reorder/2(time) -> time/1

== system Boat_sim_HeadingHold/Subsystem/Autonomous Controller/Throttle Command/Mux Everything/Build speed command ==
  CC : Inport  OutDataType=sfix(16)  OutScaling=2^0
  Constant : Constant  OutDataTypeMode=uint8  OutDataType=sfix(16)  OutScaling=2^0  OutDataTypeStr=uint8
  Constant1 : Constant  Value=0  OutDataTypeMode=uint8  OutDataType=sfix(16)  OutScaling=2^0  OutDataTypeStr=uint8
  Constant2 : Constant  Value=0  OutDataTypeMode=uint8  OutDataType=sfix(16)  OutScaling=2^0  OutDataTypeStr=uint8
  Constant3 : Constant  Value=5  OutDataTypeMode=uint8  OutDataType=sfix(16)  OutScaling=2^0  OutDataTypeStr=uint8
  Mux : Mux  Inputs=5
  uint16 to uchar : Subsystem  AncestorBlock=uSimLib/Conversions/uint16 to uchar
  msg : Outport  OutDataType=sfix(16)  OutScaling=2^0
  wires:
  uint16 to uchar/1(uchar) -> Mux/3
  Constant/1 -> Mux/1
  Constant3/1 -> Mux/2
  Mux/1 -> msg/1
  Constant1/1 -> Mux/4
  Constant2/1 -> Mux/5
  CC/1 -> uint16 to uchar/1(ushort)

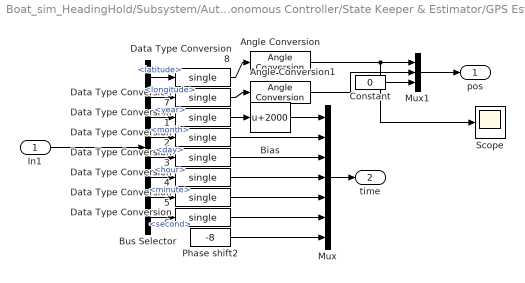
== system Boat_sim_HeadingHold/Subsystem/Autonomous Controller/State Keeper & Estimator/GPS Estimator/Subsystem/Reorder ==
  In1 : Inport
  Angle Conversion : uSimLib/Conversions/Angle Conversion  SystemSampleTime=-1  iu=deg  ou=rad
  Angle Conversion1 : uSimLib/Conversions/Angle Conversion  SystemSampleTime=-1  iu=deg  ou=rad
  Bias : Bias  Bias=2000
  Bus Selector : BusSelector  OutputSignals=latitude,longitude,year,month,day,hour,minute,second
  Constant : Constant  Value=0  OutDataTypeMode=single  OutDataType=fixdt(1, 16)  OutScaling=2^0  OutDataTypeStr=single
  Data Type Conversion{1..8} (8 alike) : DataTypeConversion  OutDataTypeMode=single  OutDataType=fixdt(1, 16)  OutScaling=2^0  OutDataTypeStr=single
  Mux : Mux  Inputs=7
  Mux1 : Mux  Inputs=3
  Phase shift2 : Constant  Value=-8  OutDataTypeMode=single  OutDataType=sfix(16)  OutScaling=2^0  OutDataTypeStr=single
  Scope : Scope
  pos : Outport
  time : Outport  Port=2
  wires:
  Bus Selector/1 -> Data Type Conversion8/1  "<latitude>"
  Bus Selector/2 -> Data Type Conversion7/1  "<longitude>"
  Data Type Conversion1/1 -> Bias/1
  Bias/1 -> Mux/1
  Data Type Conversion2/1 -> Mux/2
  Bus Selector/3 -> Data Type Conversion1/1  "<year>"
  Bus Selector/4 -> Data Type Conversion2/1  "<month>"
  Bus Selector/5 -> Data Type Conversion3/1  "<day>"
  Bus Selector/6 -> Data Type Conversion4/1  "<hour>"
  Bus Selector/7 -> Data Type Conversion5/1  "<minute>"
  Bus Selector/8 -> Data Type Conversion6/1  "<second>"
  Data Type Conversion3/1 -> Mux/3
  Data Type Conversion4/1 -> Mux/4
  Data Type Conversion5/1 -> Mux/5
  Data Type Conversion6/1 -> Mux/6
  Phase shift2/1 -> Mux/7
  In1/1 -> Bus Selector/1
  Mux/1 -> time/1
  Angle Conversion/1 -> Scope/1, Mux1/1
  Angle Conversion1/1 -> Mux1/2
  Constant/1 -> Mux1/3
  Mux1/1 -> pos/1
  Data Type Conversion7/1 -> Angle Conversion1/1
  Data Type Conversion8/1 -> Angle Conversion/1

== system Boat_sim_HeadingHold/Subsystem/Autonomous Controller/Throttle Command/Mux Everything/Build speed command/uint16 to uchar ==
  ushort : Inport
  Data Type Conversion : DataTypeConversion  OutDataTypeMode=uint16  OutDataType=fixdt(1, 16)  OutScaling=2^0  OutDataTypeStr=uint16  ConvertRealWorld=Stored Integer (SI)  RndMeth=Simplest
  Extract Bits1 : simulink/Logic and Bit Operations/Extract Bits  SystemSampleTime=-1  bitsToExtract=Upper half  numBits=8  bitIdxRange=[0 7]  outScalingMode=Treat bit field as an integer
  Extract Bits2 : simulink/Logic and Bit Operations/Extract Bits  SystemSampleTime=-1  bitsToExtract=Lower half  numBits=8  bitIdxRange=[0 7]  outScalingMode=Treat bit field as an integer
  Mux : Mux  Inputs=2
  uchar : Outport  OutDataType=fixdt(1, 16)  OutScaling=2^0
  wires:
  Mux/1 -> uchar/1
  Extract Bits2/1 -> Mux/2
  Extract Bits1/1 -> Mux/1
  ushort/1 -> Data Type Conversion/1
  Data Type Conversion/1 -> Extract Bits1/1, Extract Bits2/1

== matlab function HIL Interface/Build HIL sentence/Pack ==
  data: a input double; y output double; b input double; c input double; d input double; e input double; f input double
function y = fcn(a, b, c, d, e, f)
%#eml

y = zeros(46, 1, 'uint8');
y(1) = a;
y(2) = b;
y(3:43) = c;
y(44) = d;
y(45) = e;
y(46) = f;

== matlab function Plant/Get GPS/Embedded MATLAB Function1 ==
  data: cog output double; Vn input double; Ve input double
function cog = getCOG(Vn, Ve)
% This block supports an embeddable subset of the MATLAB language.
% See the help menu for details. 

cog = atan2(Vn,Ve);
if cog < 0;
    cog = cog + 2*pi;
end

== matlab function Subsystem/Autonomous Controller/State Keeper & Estimator/GPS Estimator/Calculate local position via velocity integral between true GPS updates ==
  data: latLonAlt input single size=[3 1]; localPosition output single; newData input boolean size=1; reset input boolean size=1; resetIntegrator output boolean size=1
function [localPosition,resetIntegrator] = estimateGPS(latLonAlt, newData, reset)
%#eml
% INPUTS:
% latLonAlt - the latitude, longitude, and altitude of the vehicle from GPS
% newData - A boolean signal specifying whether latLonAlt holds new data
% reset - A global reset boolean trigger.

% OUTPUTS:
% localPosition is the local position of the vehicle in relation to a recorded
% starting location in North-East-Down coordinates.
% resetIntegrator will reset the velocity integrator that's calculating the
% local position in between GPS reads.

persistent startingPosition lastKnownPosition newDataCounter;

% Reset everything on first startup or when a global reset is triggered
if isempty(startingPosition) || reset
    startingPosition = zeros(3, 1, 'single');
end
if isempty(lastKnownPosition) || reset
    lastKnownPosition = zeros(3, 1, 'single');
end
if isempty(newDataCounter) || reset
    newDataCounter = zeros(1, 1, 'uint8');
end

% Reset the integrator if a global reset is called
if reset
    resetIntegrator = true;
else
    resetIntegrator = false;
end

% Wait for 5 valid GPS inputs before latching a starting point
if newDataCounter < 5
    % Check that we have valid data before latching it.
    if newData && latLonAlt(1) ~= 0 && latLonAlt(2) ~= 0
        newDataCounter = newDataCounter + 1;
        startingPosition = latLonAlt;
    end
    
    % We output all 0s while we're waiting
    localPosition = zeros(3, 1, 'single');
else
    % Latch a new position if one's been received. Also reset the integrator
    % for this timestep as we have a "truth" position now.
    if newData
        lastKnownPosition = latLonAlt;
        resetIntegrator = true;
    end
    
    % Calculate the difference between the starting position and the last
    % known position.
    localPosition = dg2lg(startingPosition, latLonAlt);
end

% Not certain how this works or where I got it from.
function out = dg2lg(u1, u2)

dlat = (u2(1) - u1(1))*pi/180;
dlon = (u2(2) - u1(2))*pi/180;
lat = u1(1)*pi/180;
h = u2(3);
a = 6378137;
e2 = 0.00669437999014;

v=a./sqrt(1-e2.*sin(lat).^2);
r=v.*(1-e2)./(1-e2.*sin(lat).^2);
dx=dlat.*(r+h);
dy=dlon.*cos(lat).*(v+h);

% Map into North-East-Down coordinates
out = [dx; dy; 0];

== matlab function HIL Interface/Parse HIL input/Embedded MATLAB Function ==
  data: successCount output double; failCount output double; in input uint8; out output uint8 size=27; new output double
function [successCount, failCount, out, new] = parseMessage(in)
    persistent actuatorMessage internalSuccessCount internalFailCount;
    
    if isempty(actuatorMessage)
        actuatorMessage = zeros(27, 1, 'uint8');
        internalSuccessCount = uint32(0);
        internalFailCount = uint32(0);
    end
    
    for i = 1:size(in,1)
        [new fail data] = buildAndCheckMessage(in(i));
        if new
            actuatorMessage = data;
            internalSuccessCount = internalSuccessCount + 1;
        elseif fail
            internalFailCount = internalFailCount + 1;
        end
    end
    successCount = internalSuccessCount;
    failCount = internalFailCount;
    out = actuatorMessage;
end

function [new fail data] = buildAndCheckMessage(characterIn)
%#eml

    persistent message messageIndex messageState actuatorData;

    if isempty(message)
        message = zeros(34, 1, 'uint8');
        messageIndex = uint8(0);
        messageState = uint8(0);
        actuatorData = zeros(27, 1, 'uint8');
    end

    % This contains the function's state of whether
    % it is currently building a message.
    % 0 - Awaiting header byte 0 (%)
    % 1 - Awaiting header byte 1 (&)
    % 2 - Building message
    % 3 - Awaiting header byte 0 (^)
    % 4 - Awaiting header byte 1 (&)
    % 5 - Reading checksum character

    new = false;
    fail = false;

    % We start recording a new message if we see the header
    if messageState == 0
        if characterIn == '%'
            message(1) = characterIn;
            messageIndex = uint8(2);
            messageState = uint8(1);
        else
            fail = true;
        end
    elseif messageState == 1
        % If we don't find the necessary ampersand we start over
        % waiting for a new sentence
        if characterIn == '&'
            message(2) = characterIn;
            messageIndex = messageIndex + 1;
            messageState = uint8(2);
        elseif characterIn ~= '%'
            messageIndex = uint8(1);
            messageState = uint8(0);
            fail = true;
        end
    elseif messageState == 2
        % Record every character that comes in now that we're building a sentence.
        % Only stop if we run out of room or an asterisk is found.
        message(messageIndex) = characterIn;
        messageIndex = messageIndex + 1;
        if messageIndex > 4 && message(4) < 249 && messageIndex == message(4) + 6
            if characterIn == '^'
                messageState = uint8(3);
            else
                messageState = uint8(0);
                messageIndex = uint8(1);
                fail = true;
            end
        elseif messageIndex == length(message) - 1
            % If we've filled up the buffer, ignore the entire message as we can't store it all
            messageIndex = uint8(1);
            messageState = uint8(0);
            fail = true;
        end
    elseif messageState == 3
        % If we don't find the necessary ampersand we continue
        % recording data as we haven't found the footer yet until
        % we've filled up the entire message (ends at 124 characters
        % as we need room for the 2 footer chars).
        message(messageIndex) = characterIn;
        messageIndex = messageIndex + 1;
        if characterIn == '&'
            messageState = uint8(4);
        elseif messageIndex == length(message)
            messageState = uint8(0);
            messageIndex = uint8(1);
            fail = true;
        end
    elseif messageState == 4
        % Record the checksum byte.
        message(messageIndex) = characterIn;

        % The checksum is now verified and if successful the message
        % is stored in the appropriate struct.
        checksumCalculated = uint8(0);
        for i=3:messageIndex-3
            checksumCalculated = bitxor(checksumCalculated, message(i));
        end

        if message(messageIndex) == checksumCalculated
            % If we've found an actuator message, update our local data store
            if message(3) == 2
                actuatorData = message(5:31);
                new = true;
            end
        else
            fail = true;
        end

        % We clear all state variables here regardless of success.
        messageIndex = uint8(1);
        messageState = uint8(0);
        message = zeros(34,1,'uint8');
    end

    data = actuatorData;
end

== matlab function Plant/Actuator Dynamics/Embedded MATLAB Function ==
  data: trigger input double; angle output double; direction input double; reset input double; resetToAngle input double
function angle = fcn(trigger, direction, reset, resetToAngle)
%#eml

% Keep a variable for tracking the rudder angle internally
persistent integratedAngle;
if isempty(integratedAngle)
    integratedAngle = single(0.0);
end

% Update the rudder angle given a reset
if reset
    integratedAngle = resetToAngle;
end

% If a trigger signal is received, increment the rudder 0.005rads in the
% proper direction. This is only done if the rudder hasn't reached the
% 45deg limit yet though.
if trigger
    if direction == 0 && integratedAngle > -0.785
        integratedAngle = integratedAngle - 0.005;
    elseif direction == 1 && integratedAngle < 0.785
        integratedAngle = integratedAngle + 0.005;
    end
end

% Finally output the calculated angle
angle = integratedAngle;

== matlab function Subsystem/Autonomous Controller/Rudder Command/Latch first signal ==
  data: haveHeading output double; heading input single size=1; latchedHeading output single size=1; reset input boolean size=1
function [haveHeading,latchedHeading] = latchFirstHeading(heading, reset)
%#eml

% This Matlab function latches its input and only resets it when a reset is triggered.

persistent storedHeading haveData;

% Reset everything on first startup or when a global reset is triggered
if isempty(storedHeading) || reset
    storedHeading = single(0);
    haveData = false;
end

if ~haveData && ~reset
    storedHeading = heading;
    haveData = true;
end

haveHeading = haveData;
latchedHeading = storedHeading;

== matlab function Subsystem/Select current waypoint track ==
  data: reset output double; nextTrack input double; resetTrackNumber input double; test_waypoints parameter double; figure8_waypoints parameter double; sampling_waypoints parameter double; waypoints output double
function [reset, waypoints] = selectTrack(nextTrack, resetTrackNumber, test_waypoints, figure8_waypoints, sampling_waypoints)
%#eml


% Initialize trackNumber.
% This variable is our state, which is the set of waypoints we're navigating
% between.
persistent trackNumber;
if isempty(trackNumber)
    trackNumber = uint8(1);
end

% Here is the logic for switching tracks. trackReset resets the trackNumber
% and nextTrack increments the track number
if resetTrackNumber
    trackNumber = uint8(1);
    reset = true;
elseif nextTrack
    trackNumber = trackNumber + uint8(1);
    if trackNumber > 3
        trackNumber = uint8(1);
    end
    reset = true;
else
    reset = false;
end

% 1 is for the test waypoints, 2 is for the figure eight, and 3 is
% for the data gathering waypoints.
switch trackNumber
    case 1
        waypoints = test_waypoints;
    case 2
        waypoints = figure8_waypoints;
    case 3
        waypoints = sampling_waypoints;
    otherwise
        waypoints = zeros(size(test_waypoints), 'int32');
end

== matlab function HIL Interface/Parse HIL input/Unpack sensor data ==
  data: u input uint8; rudderEnable output double; rudderDirection output double; rudderUp output double; rudderPeriod output double; ballastEnable output double; ballastDirection output double; throttleIdentifier output double; throttleData output double; throttleSize output double; throttleTrigger output double; timestamp output double; rudderAngle output double; sensorOverride output double
function [rudderEnable, rudderDirection, rudderUp, rudderPeriod, ballastEnable, ballastDirection, throttleIdentifier, throttleData, throttleSize, throttleTrigger, timestamp, rudderAngle, sensorOverride] = unpack(u)
%#eml

rudderEnable = u(1);
rudderDirection = u(2);
rudderUp = typecast(u(3:4), 'uint16');
rudderPeriod = typecast(u(5:6), 'uint16');
ballastEnable = u(7);
ballastDirection = u(8);
throttleIdentifier = typecast(u(9:12), 'uint32');
throttleData = u(13:18);
throttleSize = u(19);
throttleTrigger = u(20);
timestamp = typecast(u(21:22), 'uint16');
rudderAngle = typecast(u(23:26), 'single');
sensorOverride = u(27);

== matlab function HIL Interface/Pack ==
  data: speed input double; lat input double; lon input double; alt input double; yr input double; mon input double; day input double; hr input double; min input double; sec input double; cog input double; sog input double; newData input double; y output double; rudderPosition input double; rudderStarboardLimit input double; rudderPortLimit input double; ballastPosition input double; ballastStarboardLimit input double; ballastPortLimit input double; timestamp input double
function y = u(speed, lat, lon, alt, yr, mon, day, hr, min, sec, cog, sog, newData, rudderPosition, rudderStarboardLimit, rudderPortLimit, ballastPosition, ballastStarboardLimit, ballastPortLimit, timestamp)
%#eml

y = zeros(39, 1, 'uint8');
y(1:2) = typecast(speed, 'uint8');
y(3:6) = typecast(lat, 'uint8');
y(7:10) = typecast(lon, 'uint8');
y(11:14) = typecast(alt, 'uint8');
y(15) = yr;
y(16) = mon;
y(17) = day;
y(18) = hr;
y(19) = min;
y(20) = sec;
y(21:24) = typecast(cog, 'uint8');
y(25:28) = typecast(sog, 'uint8');
y(29) = newData;
y(30:31) = typecast(rudderPosition, 'uint8');
y(32) = rudderStarboardLimit;
y(33) = rudderPortLimit;
y(34:35) = typecast(ballastPosition, 'uint8');
y(36) = ballastStarboardLimit;
y(37) = ballastPortLimit;
y(38:39) = typecast(timestamp, 'uint8');

== matlab function HIL Interface/Parse HIL input/Embedded MATLAB Function2 ==
  data: u1 input double; y output double; u2 input double
function y = safeDiv(u1, u2)
%#eml

if u2 == 0
    y = u1;
else
    y = u1 / u2;
end

== matlab function Subsystem/Autonomous Controller/Throttle Command/Mux Everything/Select data packet ==
  data: y output double; dis input double; en input double
function y = fcn(dis, en)
% This block controls the switch selecting between enable, 
% disable, and speed commands. If disable and enable are
% both set high, disable overrides anything else.

y = uint8(3);
if dis == 1
    y = uint8(1);
elseif en == 1
    y = uint8(2);
end
